simulink model "stateFeedback_closedLoop"  (R2020b)
settings: Solver=FixedStepAuto  StartTime=0.0  StopTime=70  FixedStep=dt  RelTol=1e-3
values from neighbouring files (symbols this model uses):
  A = double(sModelWeights.A)    [extract_model_params_from_python.m]
  A_bla = sBLA.A    [extract_model_params_from_python.m]
  B = double(sModelWeights.Bu)    [extract_model_params_from_python.m]
  B_bla = sBLA.B(:, 1:nu)    [extract_model_params_from_python.m]
  C = double(sModelWeights.C)    [extract_model_params_from_python.m]
  C_bla = sBLA.C    [extract_model_params_from_python.m]
  dcg = dcgain(sys_cl)    [closedLoopresults_pendulum.m]
  dcg_bla = dcgain(sys_bla_cl)    [closedLoopresults_pendulum.m]
  dt = 0.1    [closedLoopresults_pendulum.m]    (also in test_unitaire.m)
  f = 3    [closedLoopresults_pendulum.m]
  g = 9.81    [closedLoopresults_pendulum.m]
  G = double(sModelWeights.Bd)    [extract_model_params_from_python.m]
  G_bla = sBLA.B(:,nu+1:nu+np)    [extract_model_params_from_python.m]
  K = place(A,B,e_cl)    [closedLoopresults_pendulum.m]
  K_bla = place(A_bla, B_bla, e_cl)    [closedLoopresults_pendulum.m]
  l = 1    [closedLoopresults_pendulum.m]
  L = place(A',C',eAo)'    [closedLoopresults_pendulum.m]
  L_bla = place(A_bla',C_bla',eAo_bla)'    [closedLoopresults_pendulum.m]
  m = 2    [closedLoopresults_pendulum.m]
  np = net_dims(2)    [load_workspace.m]    (also in test_unitaire.m = 1)
  nu = net_dims(1)    [load_workspace.m]    (also in test_unitaire.m = 1)
  nx = 2    [closedLoopresults_pendulum.m]    (also in load_workspace.m = net_dims(3); test_unitaire.m)
  theta0 = 0    [closedLoopresults_pendulum.m]
  W_out = double(sModelWeights.alpha_out)    [extract_model_params_from_python.m]
  W_p_in = double(sModelWeights.alpha_in_d)    [extract_model_params_from_python.m]
  W_y_in = double(sModelWeights.alpha_in_y)    [extract_model_params_from_python.m]
undefined symbols (not defined in the file or in its folder): b_in, b_out
settings Model: Creator=MT  LastModifiedBy=alexandre
settings DebuggingCC: UnconnectedInputMsg=none  UnconnectedOutputMsg=none  UnconnectedLineMsg=none  SFMachineParentedDataDiag=error  ArithmeticOperatorsInVariantConditions=warning
settings SFSimCC: CustomCodeUndefinedFunction=UseInterfaceOnly

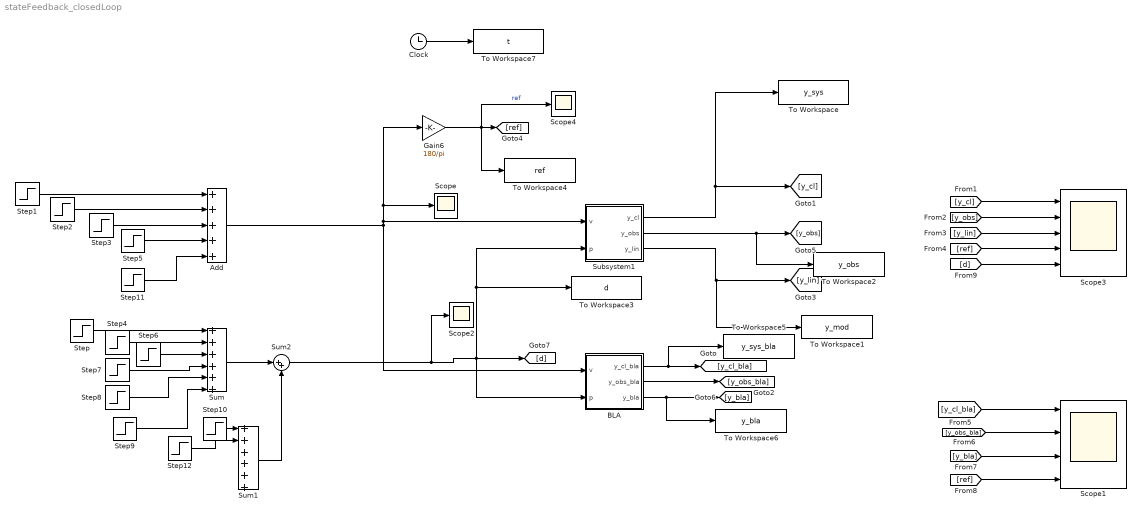
== system stateFeedback_closedLoop ==
  Add : Sum  Inputs=+++++
  BLA : Subsystem
  Clock : Clock
  Gain6 : Gain  Gain=180/pi
  Scope : Scope
  Scope1 : Scope  NumInputPorts=4
  Scope2 : Scope
  Scope3 : Scope  NumInputPorts=5
  Scope4 : Scope
  Step : Step  Time=10  After=5  SampleTime=0
  Step1 : Step  After=pi/2.5  SampleTime=0
  Step10 : Step  Time=40  After=-4  SampleTime=0
  Step11 : Step  Time=45  After=-pi/4  SampleTime=0
  Step12 : Step  Time=45  After=-4  SampleTime=0
  Step2 : Step  Time=5  After=-pi/2.5  SampleTime=0
  Step3 : Step  Time=10  After=pi/4  SampleTime=0
  Step4 : Step  Time=15  After=-8  SampleTime=0
  Step5 : Step  Time=40  After=-pi/4  SampleTime=0
  Step6 : Step  Time=20  After=3  SampleTime=0
  Step7 : Step  Time=25  After=5  SampleTime=0
  Step8 : Step  Time=30  After=5  SampleTime=0
  Step9 : Step  Time=35  After=-5  SampleTime=0
  Subsystem1 : Subsystem
  Sum : Sum  Inputs=++++++
  Sum1 : Sum  Inputs=++++++
  Sum2 : Sum  Inputs=|++
  To Workspace : ToWorkspace  VariableName=y_sys  SampleTime=dt
  To Workspace1 : ToWorkspace  VariableName=y_mod  SampleTime=dt
  To Workspace2 : ToWorkspace  VariableName=y_obs  SampleTime=dt
  To Workspace3 : ToWorkspace  VariableName=d  SampleTime=dt
  To Workspace4 : ToWorkspace  VariableName=ref  SampleTime=dt
  To Workspace5 : ToWorkspace  VariableName=y_sys_bla  SampleTime=dt
  To Workspace6 : ToWorkspace  VariableName=y_bla  SampleTime=dt
  To Workspace7 : ToWorkspace  VariableName=t  SampleTime=dt
  wires:
  Step1/1 -> Add/1
  Step2/1 -> Add/2
  Step3/1 -> Add/3
  Add/1 -> BLA/1(v), Subsystem1/1(v), Gain6/1, Scope/1
  [y_cl] -> Scope3/1
  [y_obs] -> Scope3/2
  [y_lin] -> Scope3/3
  [ref] -> Scope3/4
  Subsystem1/1(y_cl) -> To Workspace/1, [y_cl]
  Subsystem1/2(y_obs) -> To Workspace2/1, [y_obs]
  Subsystem1/3(y_lin) -> To Workspace1/1, [y_lin]
  [y_cl_bla] -> Scope1/1
  [ref] -> Scope1/4
  [y_bla] -> Scope1/3
  [y_obs_bla] -> Scope1/2
  BLA/1(y_cl_bla) -> To Workspace5/1, [y_cl_bla]
  BLA/2(y_obs_bla) -> [y_obs_bla]
  BLA/3(y_bla) -> To Workspace6/1, [y_bla]
  Step/1 -> Sum/1
  Step4/1 -> Sum/2
  [d] -> Scope3/5
  Gain6/1 -> Scope4/1, To Workspace4/1, [ref]  "ref"
  Step6/1 -> Sum/3
  Clock/1 -> To Workspace7/1
  Step7/1 -> Sum/4
  Step8/1 -> Sum/5
  Step9/1 -> Sum/6
  Step5/1 -> Add/4
  Sum/1 -> Sum2/1
  Sum1/1 -> Sum2/2
  Sum2/1 -> Scope2/1, BLA/2(p), Subsystem1/2(p), To Workspace3/1, [d]
  Step10/1 -> Sum1/1
  Step11/1 -> Add/5
  Step12/1 -> Sum1/2

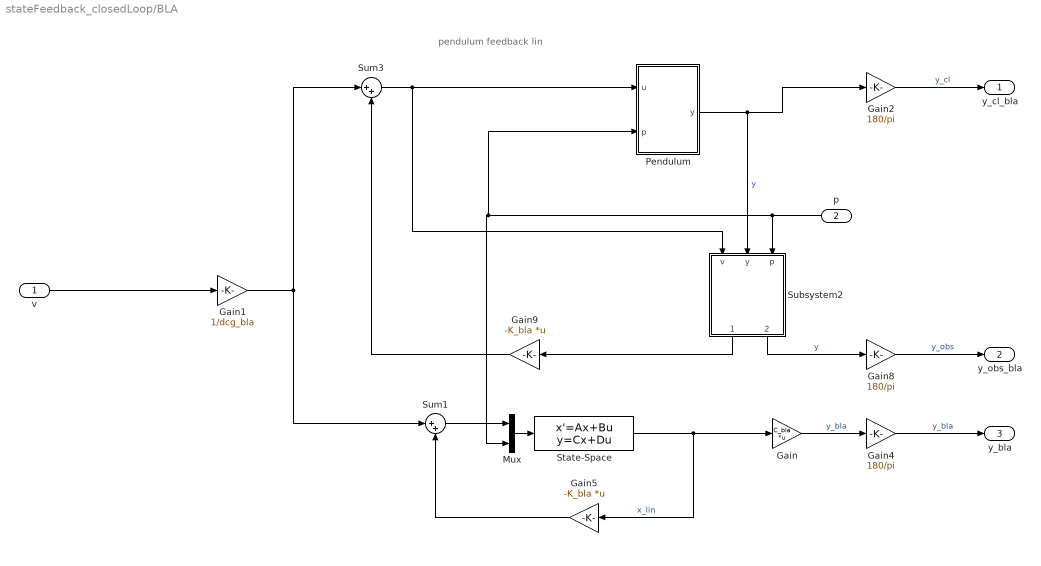
== system stateFeedback_closedLoop/BLA ==
  note: pendulum feedback lin
  v : Inport
  p : Inport  Port=2
  Gain : Gain  Gain=C_bla  Multiplication=Matrix(K*u) (u vector)
  Gain1 : Gain  Gain=1/dcg_bla
  Gain2 : Gain  Gain=180/pi
  Gain4 : Gain  Gain=180/pi
  Gain5 : Gain  Gain=-K_bla  Multiplication=Matrix(K*u) (u vector)
  Gain8 : Gain  Gain=180/pi
  Gain9 : Gain  Gain=-K_bla  Multiplication=Matrix(K*u) (u vector)
  Mux : Mux  Inputs=2
  Pendulum : Subsystem
  State-Space : StateSpace  A=A_bla  B=[B_bla, G_bla]  C=eye(nx)  D=zeros(nx, nu+np)  InitialCondition=0
  Subsystem2 : Subsystem
  Sum1 : Sum  Inputs=|++
  Sum3 : Sum  Inputs=|++
  y_cl_bla : Outport
  y_obs_bla : Outport  Port=2
  y_bla : Outport  Port=3
  wires:
  Gain4/1 -> y_bla/1  "y_bla"
  Gain2/1 -> y_cl_bla/1  "y_cl"
  State-Space/1 -> Gain5/1, Gain/1  "x_lin"
  Gain5/1 -> Sum1/2
  Gain/1 -> Gain4/1  "y_bla"
  Gain8/1 -> y_obs_bla/1  "y_obs"
  Gain9/1 -> Sum3/2
  Subsystem2/2(y_hat_out) -> Gain8/1  "y"
  Gain1/1 -> Sum3/1, Sum1/1
  v/1 -> Gain1/1
  Subsystem2/1(x_hat_out) -> Gain9/1
  Sum3/1 -> Pendulum/1(u), Subsystem2/1(v)
  p/1 -> Pendulum/2(p), Mux/2, Subsystem2/3(p)
  Mux/1 -> State-Space/1
  Sum1/1 -> Mux/1
  Pendulum/1(y) -> Subsystem2/2(y), Gain2/1  "y"

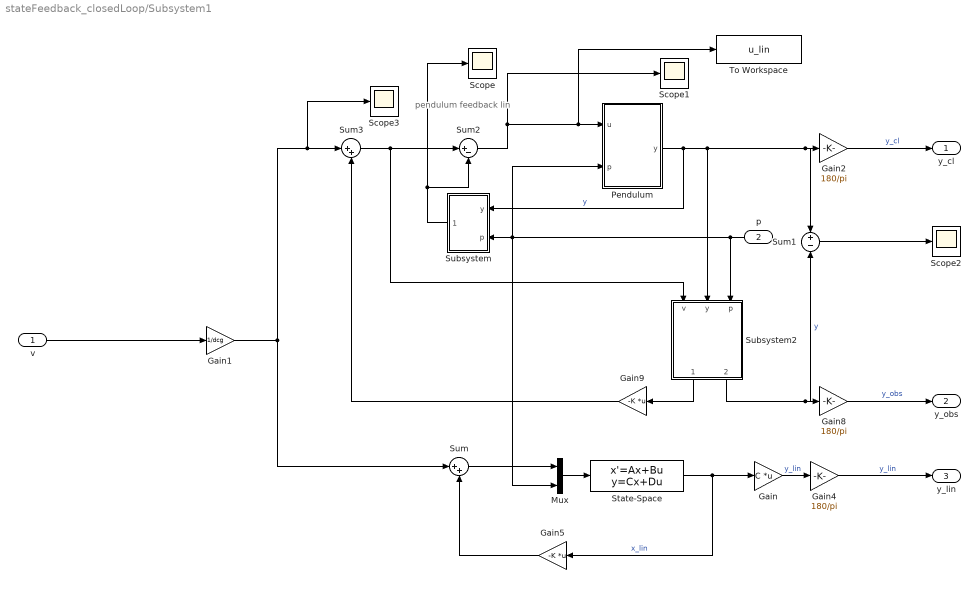
== system stateFeedback_closedLoop/Subsystem1 ==
  note: pendulum feedback lin
  v : Inport
  p : Inport  Port=2
  Gain : Gain  Gain=C  Multiplication=Matrix(K*u) (u vector)
  Gain1 : Gain  Gain=1/dcg
  Gain2 : Gain  Gain=180/pi
  Gain4 : Gain  Gain=180/pi
  Gain5 : Gain  Gain=-K  Multiplication=Matrix(K*u) (u vector)
  Gain8 : Gain  Gain=180/pi
  Gain9 : Gain  Gain=-K  Multiplication=Matrix(K*u) (u vector)
  Mux : Mux  Inputs=2
  Pendulum : Subsystem
  Scope{,1..3} (4 alike) : Scope
  State-Space : StateSpace  A=A  B=[B, G]  C=eye(nx)  D=zeros(nx, nu+np)  InitialCondition=0
  Subsystem : Subsystem
  Subsystem2 : Subsystem
  Sum : Sum  Inputs=|++
  Sum1 : Sum  Inputs=+-
  Sum2 : Sum  Inputs=|+-
  Sum3 : Sum  Inputs=|++
  To Workspace : ToWorkspace  VariableName=u_lin  SampleTime=dt
  y_cl : Outport
  y_obs : Outport  Port=2
  y_lin : Outport  Port=3
  wires:
  Gain4/1 -> y_lin/1  "y_lin"
  Gain2/1 -> y_cl/1  "y_cl"
  State-Space/1 -> Gain5/1, Gain/1  "x_lin"
  Gain/1 -> Gain4/1  "y_lin"
  Gain8/1 -> y_obs/1  "y_obs"
  Gain9/1 -> Sum3/2
  Subsystem/1(f_yp) -> Sum2/2, Scope/1
  Subsystem2/2(y_hat_out) -> Sum1/2, Gain8/1  "y"
  p/1 -> Subsystem2/3(p), Pendulum/2(p), Mux/2, Subsystem/2(p)
  Gain1/1 -> Scope3/1, Sum3/1, Sum/1
  v/1 -> Gain1/1
  Sum3/1 -> Sum2/1, Subsystem2/1(v)
  Pendulum/1(y) -> Subsystem/1(y), Sum1/1, Gain2/1, Subsystem2/2(y)  "y"
  Subsystem2/1(x_hat_out) -> Gain9/1
  Sum2/1 -> Scope1/1, To Workspace/1, Pendulum/1(u)
  Mux/1 -> State-Space/1
  Sum/1 -> Mux/1
  Gain5/1 -> Sum/2
  Sum1/1 -> Scope2/1

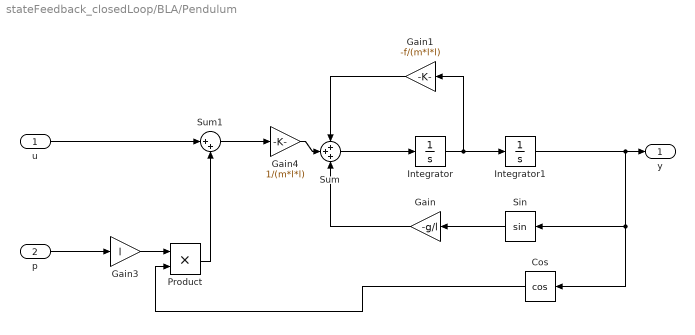
== system stateFeedback_closedLoop/BLA/Pendulum ==
  u : Inport
  p : Inport  Port=2
  Cos : Trigonometry  Operator=cos
  Gain : Gain  Gain=-g/l
  Gain1 : Gain  Gain=-f/(m*l*l)
  Gain3 : Gain  Gain=l
  Gain4 : Gain  Gain=1/(m*l*l)
  Integrator : Integrator
  Integrator1 : Integrator  InitialCondition=theta0*pi/180
  Product : Product
  Sin : Trigonometry
  Sum : Sum  Inputs=+++
  Sum1 : Sum  Inputs=|++
  y : Outport
  wires:
  Sum1/1 -> Gain4/1
  Product/1 -> Sum1/2
  Sum/1 -> Integrator/1
  Sin/1 -> Gain/1
  p/1 -> Gain3/1
  u/1 -> Sum1/1
  Integrator/1 -> Gain1/1, Integrator1/1
  Integrator1/1 -> y/1, Cos/1, Sin/1
  Cos/1 -> Product/2
  Gain3/1 -> Product/1
  Gain1/1 -> Sum/1
  Gain4/1 -> Sum/2
  Gain/1 -> Sum/3

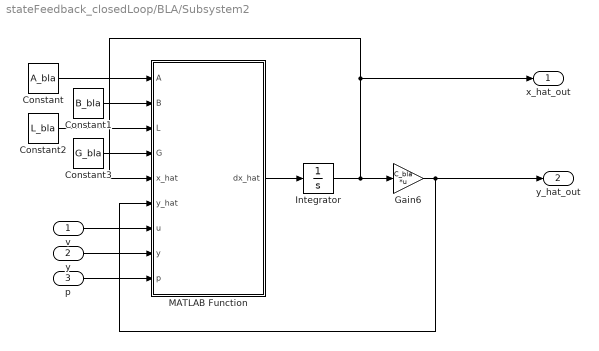
== system stateFeedback_closedLoop/BLA/Subsystem2 ==
  v : Inport
  y : Inport  Port=2
  p : Inport  Port=3
  Constant : Constant  Value=A_bla
  Constant1 : Constant  Value=B_bla
  Constant2 : Constant  Value=L_bla
  Constant3 : Constant  Value=G_bla
  Gain6 : Gain  Gain=C_bla  Multiplication=Matrix(K*u) (u vector)
  Integrator : Integrator
  MATLAB Function : MATLAB Function  TreatAsAtomicUnit=on
  x_hat_out : Outport
  y_hat_out : Outport  Port=2
  wires:
  Constant1/1 -> MATLAB Function/2(B)
  Integrator/1 -> x_hat_out/1, MATLAB Function/5(x_hat), Gain6/1
  Constant/1 -> MATLAB Function/1(A)
  MATLAB Function/1(dx_hat) -> Integrator/1
  y/1 -> MATLAB Function/8(y)
  Gain6/1 -> MATLAB Function/6(y_hat), y_hat_out/1
  Constant2/1 -> MATLAB Function/3(L)
  v/1 -> MATLAB Function/7(u)
  Constant3/1 -> MATLAB Function/4(G)
  p/1 -> MATLAB Function/9(p)

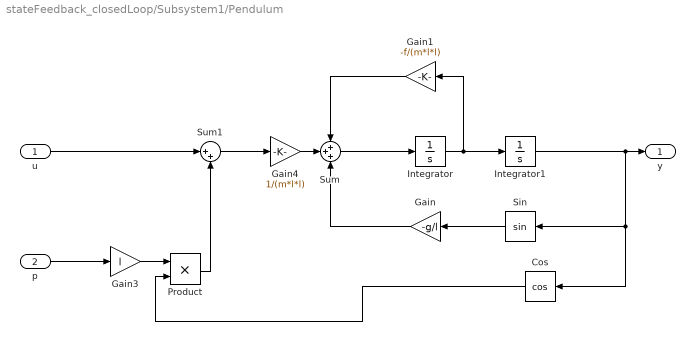
== system stateFeedback_closedLoop/Subsystem1/Pendulum ==
  u : Inport
  p : Inport  Port=2
  Cos : Trigonometry  Operator=cos
  Gain : Gain  Gain=-g/l
  Gain1 : Gain  Gain=-f/(m*l*l)
  Gain3 : Gain  Gain=l
  Gain4 : Gain  Gain=1/(m*l*l)
  Integrator : Integrator
  Integrator1 : Integrator  InitialCondition=theta0*pi/180
  Product : Product
  Sin : Trigonometry
  Sum : Sum  Inputs=+++
  Sum1 : Sum  Inputs=|++
  y : Outport
  wires:
  Sum1/1 -> Gain4/1
  Product/1 -> Sum1/2
  Sum/1 -> Integrator/1
  Sin/1 -> Gain/1
  p/1 -> Gain3/1
  u/1 -> Sum1/1
  Integrator/1 -> Gain1/1, Integrator1/1
  Integrator1/1 -> y/1, Cos/1, Sin/1
  Cos/1 -> Product/2
  Gain3/1 -> Product/1
  Gain1/1 -> Sum/1
  Gain4/1 -> Sum/2
  Gain/1 -> Sum/3

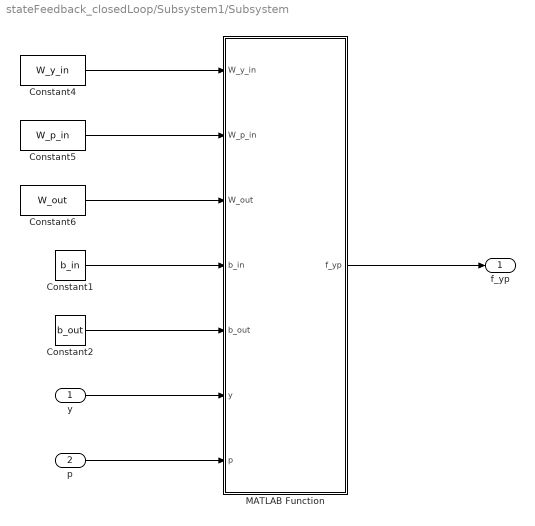
== system stateFeedback_closedLoop/Subsystem1/Subsystem ==
  y : Inport
  p : Inport  Port=2
  Constant1 : Constant  Value=b_in  VectorParams1D=off
  Constant2 : Constant  Value=b_out  VectorParams1D=off
  Constant4 : Constant  Value=W_y_in  VectorParams1D=off
  Constant5 : Constant  Value=W_p_in  VectorParams1D=off
  Constant6 : Constant  Value=W_out  VectorParams1D=off
  MATLAB Function : MATLAB Function  TreatAsAtomicUnit=on
  f_yp : Outport
  wires:
  y/1 -> MATLAB Function/6(y)
  Constant5/1 -> MATLAB Function/2(W_p_in)
  Constant4/1 -> MATLAB Function/1(W_y_in)
  Constant6/1 -> MATLAB Function/3(W_out)
  MATLAB Function/1(f_yp) -> f_yp/1
  p/1 -> MATLAB Function/7(p)
  Constant1/1 -> MATLAB Function/4(b_in)
  Constant2/1 -> MATLAB Function/5(b_out)

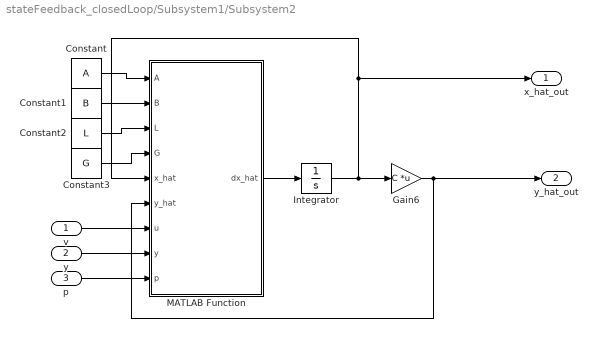
== system stateFeedback_closedLoop/Subsystem1/Subsystem2 ==
  v : Inport
  y : Inport  Port=2
  p : Inport  Port=3
  Constant : Constant  Value=A
  Constant1 : Constant  Value=B
  Constant2 : Constant  Value=L
  Constant3 : Constant  Value=G
  Gain6 : Gain  Gain=C  Multiplication=Matrix(K*u) (u vector)
  Integrator : Integrator
  MATLAB Function : MATLAB Function  TreatAsAtomicUnit=on
  x_hat_out : Outport
  y_hat_out : Outport  Port=2
  wires:
  Constant1/1 -> MATLAB Function/2(B)
  Integrator/1 -> x_hat_out/1, MATLAB Function/5(x_hat), Gain6/1
  Constant/1 -> MATLAB Function/1(A)
  MATLAB Function/1(dx_hat) -> Integrator/1
  y/1 -> MATLAB Function/8(y)
  Gain6/1 -> MATLAB Function/6(y_hat), y_hat_out/1
  Constant2/1 -> MATLAB Function/3(L)
  v/1 -> MATLAB Function/7(u)
  p/1 -> MATLAB Function/9(p)
  Constant3/1 -> MATLAB Function/4(G)

== matlab function stateFeedback_closedLoop/Subsystem1/Subsystem/MATLAB Function ==
  data: W_y_in input; W_p_in input; W_out input; b_in input; b_out input; y input; f_yp output; p input
function f_yp = fcn(W_y_in,W_p_in,W_out,b_in, b_out,y,p)

f_yp = W_out*tanh(W_y_in*y+W_p_in*p+b_in)+b_out;

== matlab function stateFeedback_closedLoop/BLA/Subsystem2/MATLAB Function ==
  data: A input; B input; L input; G input; x_hat input; y_hat input; u input; dx_hat output; y input; p input
function dx_hat = fcn(A,B,L,G,x_hat,y_hat,u,y, p)

dx_hat = A*x_hat+B*u+L*(y-y_hat) + G*p;

== matlab function stateFeedback_closedLoop/Subsystem1/Subsystem2/MATLAB Function ==
  data: A input; B input; L input; G input; x_hat input; y_hat input; u input; dx_hat output; y input; p input
function dx_hat = fcn(A,B,L,G,x_hat,y_hat,u,y,p)

dx_hat = A*x_hat+B*u+L*(y-y_hat) + G*p;
